simulink model "Comparator_Model"  (R2024b)
settings: Solver=VariableStepAuto  StartTime=0.0  StopTime=10.0  RelTol=1e-3
libraries: NSA_DEVS_SINKS x8, NSA_DEVS_MATH_OPERATIONS x6, NSA_DEVS_SOURCES x2
settings Model: Creator=david  LastModifiedBy=peter
settings RTWCC: GPUComputeCapability=3.5

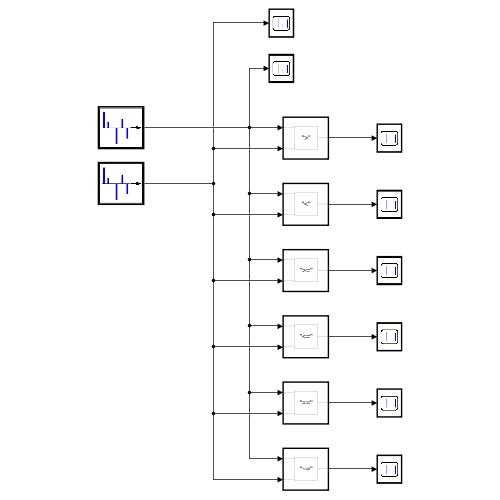
[thumbnail: Simulink's stored preview of the top-level diagram]
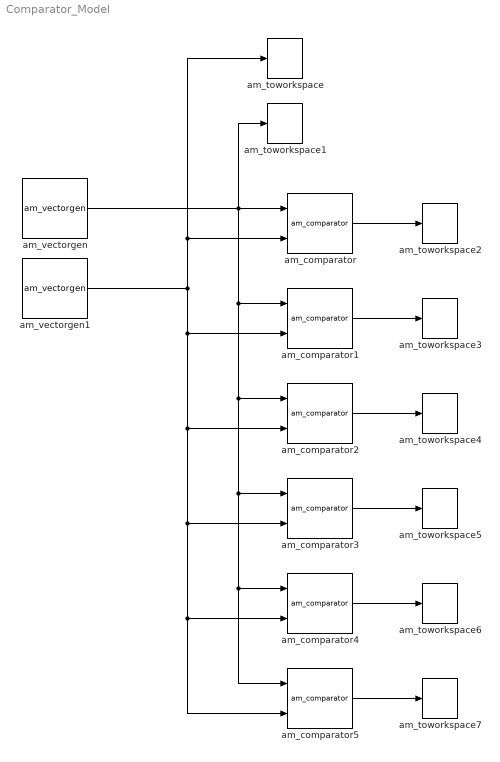
== system Comparator_Model ==
  am_comparator : NSA_DEVS_MATH_OPERATIONS/am_comparator  compop="\">\""  tau=[0,1]  debug=0
      settings: SourceProductName=Math Operations
  am_comparator1 : NSA_DEVS_MATH_OPERATIONS/am_comparator  compop="\"<\""  tau=[0,1]  debug=0
      settings: SourceProductName=Math Operations
  am_comparator2 : NSA_DEVS_MATH_OPERATIONS/am_comparator  compop="\">=\""  tau=[0,1]  debug=0
      settings: SourceProductName=Math Operations
  am_comparator3 : NSA_DEVS_MATH_OPERATIONS/am_comparator  compop="\"<=\""  tau=[0,1]  debug=0
      settings: SourceProductName=Math Operations
  am_comparator4 : NSA_DEVS_MATH_OPERATIONS/am_comparator  compop="\"==\""  tau=[0,1]  debug=0
      settings: SourceProductName=Math Operations
  am_comparator5 : NSA_DEVS_MATH_OPERATIONS/am_comparator  compop="\"~=\""  tau=[0,1]  debug=0
      settings: SourceProductName=Math Operations
  am_toworkspace : NSA_DEVS_SINKS/am_toworkspace  varname="\"genOut2\""  t0=0  format="\"vector\""  tau=[0,5]  debug=0
      settings: SourceProductName=Sinks
  am_toworkspace1 : NSA_DEVS_SINKS/am_toworkspace  varname="\"genOut1\""  t0=0  format="\"vector\""  tau=[0,5]  debug=0
      settings: SourceProductName=Sinks
  am_toworkspace2 : NSA_DEVS_SINKS/am_toworkspace  varname="\"compOut1\""  t0=0  format="\"vector\""  tau=[0,5]  debug=0
      settings: SourceProductName=Sinks
  am_toworkspace3 : NSA_DEVS_SINKS/am_toworkspace  varname="\"compOut2\""  t0=0  format="\"vector\""  tau=[0,5]  debug=0
      settings: SourceProductName=Sinks
  am_toworkspace4 : NSA_DEVS_SINKS/am_toworkspace  varname="\"compOut3\""  t0=0  format="\"vector\""  tau=[0,5]  debug=0
      settings: SourceProductName=Sinks
  am_toworkspace5 : NSA_DEVS_SINKS/am_toworkspace  varname="\"compOut4\""  t0=0  format="\"vector\""  tau=[0,5]  debug=0
      settings: SourceProductName=Sinks
  am_toworkspace6 : NSA_DEVS_SINKS/am_toworkspace  varname="\"compOut5\""  t0=0  format="\"vector\""  tau=[0,5]  debug=0
      settings: SourceProductName=Sinks
  am_toworkspace7 : NSA_DEVS_SINKS/am_toworkspace  varname="\"compOut6\""  t0=0  format="\"vector\""  tau=[0,5]  debug=0
      settings: SourceProductName=Sinks
  am_vectorgen : NSA_DEVS_SOURCES/am_vectorgen  tvec="[0, 1,  3, 7,  8,  9]"  yvec=[0, 4, -3, 2, -2, -1]  tau=[0,1]  debug=0
      settings: SourceProductName=Sources
  am_vectorgen1 : NSA_DEVS_SOURCES/am_vectorgen  tvec="[0, 1,  3, 7,  8,  9]"  yvec="[0, 2,  8, 2, -2, -9]"  tau=[0,1]  debug=0
      settings: SourceProductName=Sources
  wires:
  am_vectorgen/1 -> am_toworkspace1/1, am_comparator5/1, am_comparator4/1, am_comparator3/1, am_comparator2/1, am_comparator1/1, am_comparator/1
  am_vectorgen1/1 -> am_comparator1/2, am_comparator5/2, am_comparator4/2, am_comparator3/2, am_comparator2/2, am_toworkspace/1, am_comparator/2
  am_comparator/1 -> am_toworkspace2/1
  am_comparator1/1 -> am_toworkspace3/1
  am_comparator2/1 -> am_toworkspace4/1
  am_comparator3/1 -> am_toworkspace5/1
  am_comparator4/1 -> am_toworkspace6/1
  am_comparator5/1 -> am_toworkspace7/1
